simulink model "fig2_36_simulink"  (R2021b)
settings: Solver=ode45  StartTime=0.0  StopTime=10  RelTol=1e-3  EnableMultiTasking=on
settings Model: Creator=One Informatic  LastModifiedBy=One Informatic
settings DataIOCC: LimitDataPoints=on  SaveFormat=Array  SignalLoggingSaveFormat=ModelDataLogs  ReturnWorkspaceOutputs=off  SignalLoggingName=sigsOut
settings DebuggingCC: SaveWithParameterizedLinksMsg=none  UnderspecifiedInitializationDetection=Classic  MergeDetectMultiDrivingBlocksExec=none  SignalResolutionControl=TryResolveAllWithWarning  MultiTaskDSMMsg=warning  MultiTaskCondExecSysMsg=none
settings HardwareCC: ProdBitPerPointer=32  ProdBitPerSizeT=32  ProdBitPerPtrDiffT=32  ProdLargestAtomicFloat=None  ProdIntDivRoundTo=Undefined  ProdEndianess=Unspecified  ProdWordSize=32  ProdHWDeviceType=32-bit Generic  TargetUnknown=on
settings ModelReferenceCC: PropagateSignalLabelsOutOfModel=off
settings GRTTargetCC: CombineOutputUpdateFcns=off  GRTInterface=on
settings ConfigComp: CovMetricSettings=dw  CovSaveCumulativeToWorkspaceVar=on  CovSaveSingleToWorkspaceVar=on

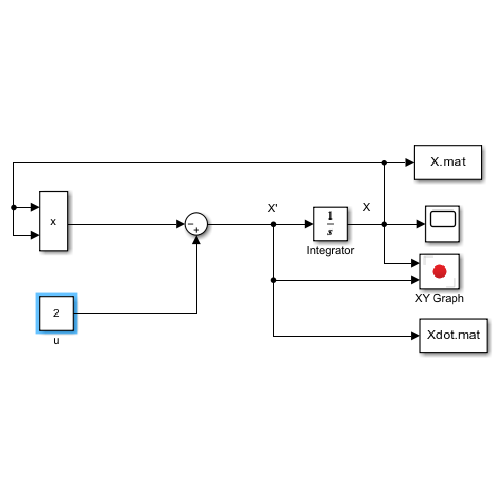
[thumbnail: Simulink's stored preview of the top-level diagram]
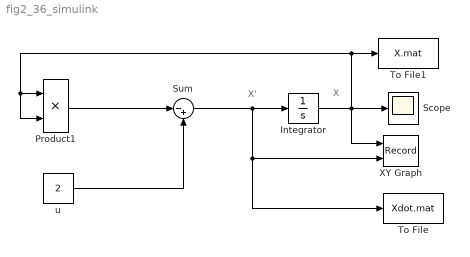
== system fig2_36_simulink ==
  note: X'
  note: X
  Integrator : Integrator  InitialCondition=-1
  Product1 : Product
  Scope : Scope
  Sum : Sum  Inputs=|-+
  To File : ToFile  Filename=Xdot.mat  MatrixName=Xdot  SampleTime=0.001
  To File1 : ToFile  Filename=X.mat  MatrixName=X  SampleTime=0.001
  XY Graph : Record  FileSettingsInternal="{\"entries\":[{\"content\":{\"excelSettings\":{\"content\":{},\"type\":\"Streamout.ExcelSettings\"}},\"type\":\"Streamout.FileSettingStorage\",\"uuid\":\"6c3b332e-3c62-4d45-88eb-e11fe2c47eab\"}],\"packageUris\":[\"http://schema.mathworks.com/mf0/streamout_blocks/R2020a\"],\"version\":\"1.0\"}"  Layout=[1 1]  SignalsInternal="{\"entries\":[{\"content\":{\"signals\":[{\"content\":{\"blockPath\":[\"fig2_36_simulink/XY Graph\"],\"channel\":[],\"dimensions\":[1],\"domain\":\"fig2_36_simulink/XY Graph\",\"lineColor\":\"#64d413\",\"plots\":[],\"port\":1,\"sid\":[\"\"],\"signalID\":116456,\"signalName\":\"Integrator\"},\"type\":\"RecordBlkView.Signal\",\"uuid\":\"e47b75ec-31e0-4925-bacc-6e560f684e42\"},{\"content\":{\"blockPath\":[\"fig2_36_simulink/XY Graph\"],\"channel\":[],\"dimensions\":[1],\"domain\":\"fig2_36_simulink/XY Graph\",\"lineColor\":\"#ff13a6\",\"plots\":[],\"port\":2,\"sid\":[\"\"],\"signalID\":116460,\"signalName\":\"Sum\"},\"type\":\"RecordBlkView.Signal\",\"uuid\":\"e2994e9c-c365-4819-bdbf-b23fd86351ca\"}]},\"type\":\"RecordBlkView.InputSignals\",\"uuid\":\"e44e69ab-035e-4559-b11f-a550568ae93a\"}],\"packageUris\":[\"http://schema.mathworks.com/mf0/streamout_blocks/R2020a\"],\"version\":\"1.0\"}"  VisualizationBindings="{\"xyplotplugin\":{\"info\":[{\"series\":[],\"subplotID\":1}]}}"  CompatibilityTag=XY
  u : Constant  Value=2
  wires:
  Product1/1 -> Sum/1
  Sum/1 -> Integrator/1, To File/1, XY Graph/2
  Integrator/1 -> To File1/1, Product1/2, Product1/1, Scope/1, XY Graph/1
  u/1 -> Sum/2
